simulink model "tester36"  (R2022b)
settings: Solver=VariableStepAuto  StartTime=0.0  StopTime=10  RelTol=1e-3
values from neighbouring files (symbols this model uses):
  IPR = 0.99    [dane.m]    (also in tester23.m; wykresownik33.m; wykresownik35.m; wykresownik36.m)
  P3tDIVP2t_perf = 1.0101    [dane.m]    (also in tester23.m = 1; wykresownik33.m = 1; wykresownik35.m = 1; wykresownik36.m = 1)
  P3tDIVP2t_safe = 1.35    [dane.m]    (also in tester23.m; wykresownik33.m; wykresownik35.m; wykresownik36.m)
libraries: fl_lib x6, nesl_utility x4, SimscapeFluids_lib x3, simulink x1
settings Model: Creator=48519  LastModifiedBy=48519
settings ModelReferenceCC: EnableRefExpFcnMdlSchedulingChecks=on

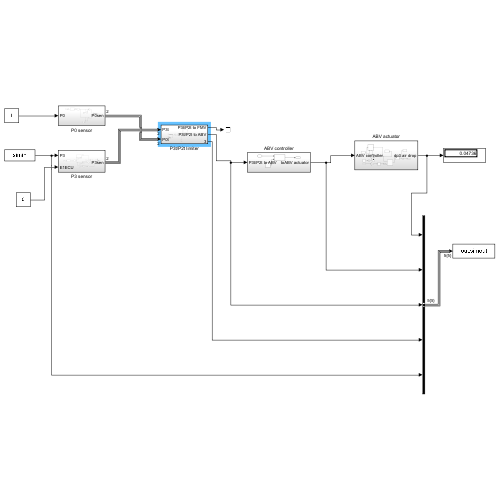
[thumbnail: Simulink's stored preview of the top-level diagram]
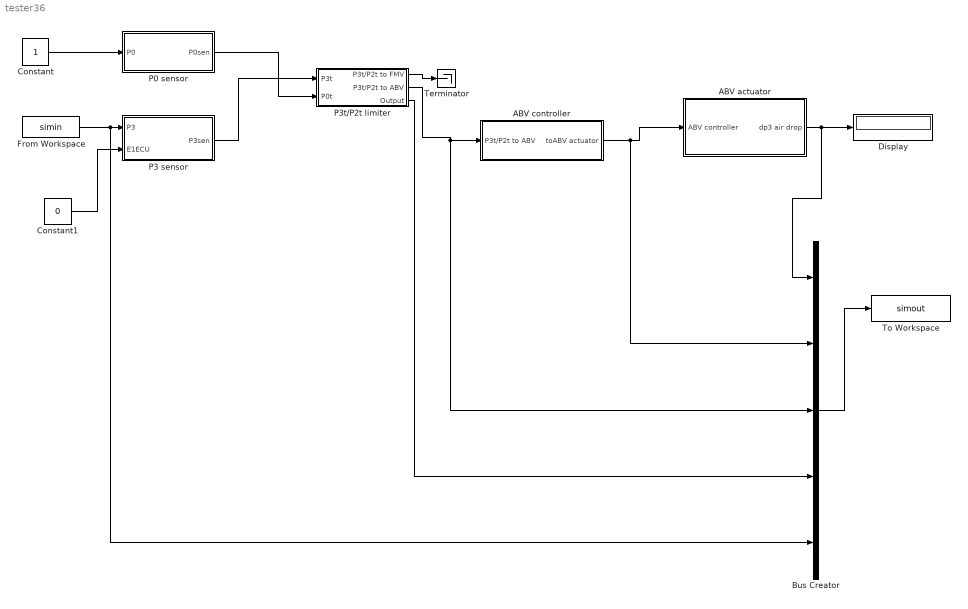
== system tester36 ==
  ABV actuator : Subsystem
  ABV controller : Subsystem
  Bus Creator : BusCreator  Inputs=5
  Constant : Constant
  Constant1 : Constant  Value=0
  Display : Display
  From Workspace : FromWorkspace  VariableName=simin
  P0 sensor : Subsystem
  P3 sensor : Subsystem
  P3t/P2t limiter : Subsystem
  Terminator : Terminator
  To Workspace : ToWorkspace  VariableName=simout  SaveFormat=Timeseries  SampleTime=-1
  wires:
  P3 sensor/1(P3sen) -> P3t/P2t limiter/1(P3t)
  P3t/P2t limiter/1(P3t/P2t to FMV) -> Terminator/1
  P3t/P2t limiter/2(P3t/P2t to ABV) -> Bus Creator/3, ABV controller/1(P3t/P2t to ABV)
  ABV actuator/1(dp3 air drop) -> Bus Creator/1, Display/1
  Constant/1 -> P0 sensor/1(P0)
  From Workspace/1 -> Bus Creator/5, P3 sensor/1(P3)
  Constant1/1 -> P3 sensor/2(E1ECU)
  Bus Creator/1 -> To Workspace/1
  ABV controller/1(toABV actuator) -> Bus Creator/2, ABV actuator/1(ABV controller)
  P3t/P2t limiter/3(Output) -> Bus Creator/4
  P0 sensor/1(P0sen) -> P3t/P2t limiter/2(P0t)

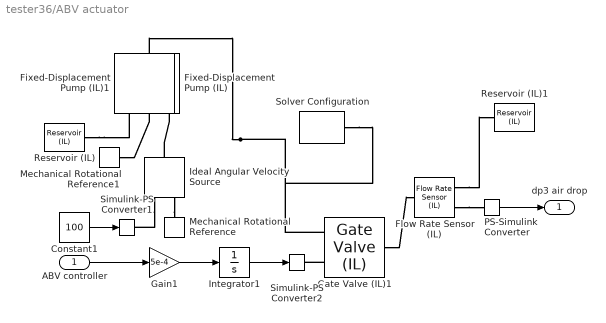
== system tester36/ABV actuator ==
  ABV controller : Inport
  Constant1 : Constant  Value=100
  Fixed-Displacement Pump (IL) : SimscapeFluids_lib/Isothermal Liquid/Pumps & Motors/Fixed-Displacement Pump (IL)  leakage_friction_spec=fluids.isothermal_liquid.pumps_motors.enum.pump_motor_loss_spec.analytical  displacement=30 cm^3/rev  omega_nominal=188 rad/s  p_nominal=10 MPa  vol_eff_nominal=0.92  mech_eff_nominal=0.88  no_load_torque=0 N*m  p_diff_eff_TLU=[.1, 1, 2] MPa  omega_eff_TLU=[25, 50, 100, 200, 300, 400] rad/s  vol_eff_TLU=[.816, .908, .954, .977, .981, .984; .325, .663, .831, .916, .925, .946; .137, .568, .78, .892, .893, .91]  mech_eff_TLU=[.996, .996, .996, .996, .996, .996; .988, .989, .989, .989, .989, .99; .981, .981, .982, .982, .983, .984]  p_diff_loss_TLU=[.1, 1, 2] MPa  omega_loss_TLU=[25, 50, 100, 200, 300, 400] rad/s  vol_loss_TLU=1e-3 * [.023, .023, .023, .023, .0285, .032; .0844, .0842, .0845, .084, .1125, .108; .1079, .108, .11, .108, .1605, .18] m^3/s  mech_loss_TLU=[.002, .002, .002, .002, .002, .002; .0607, .0556, .0556, .0556, .0556, .0505; .1937, .1937, .1833, .1833, .1729, .1626] N*m  vol_eff_min=1e-3  vol_eff_max=1  mech_eff_min=1e-3  mech_eff_max=1  pressure_threshold=1e-3 MPa  omega_threshold=10 rad/s  quadrant_check=simscape.enum.assert.action.none  pump_mode_check=simscape.enum.assert.action.none  pressure_check=simscape.enum.assert.action.none  p_min_valid=0.101325 MPa
      settings: LogSimulationData=on  InternalSimscapePortConfiguration="{\"Bottom\":[{\"id\":\"A\",\"label\":\"A\",\"type\":\"foundation.isothermal_liquid.isothermal_liquid\"}],\"Left\":[],\"Right\":[{\"id\":\"R\",\"label\":\"R\",\"type\":\"foundation.mechanical.rotational.rotational\"},{\"id\":\"C\",\"label\":\"C\",\"type\":\"foundation.mechanical.rotational.rotational\"}],\"Top\":[{\"id\":\"B\",\"label\":\"B\",\"type\":\"foundation.isothermal_liquid.isothermal_liquid\"}]}"
  Fixed-Displacement Pump (IL)1 : SimscapeFluids_lib/Isothermal Liquid/Pumps & Motors/Fixed-Displacement Pump (IL)  leakage_friction_spec=fluids.isothermal_liquid.pumps_motors.enum.pump_motor_loss_spec.analytical  displacement=30 cm^3/rev  omega_nominal=188 rad/s  p_nominal=10 MPa  vol_eff_nominal=0.92  mech_eff_nominal=0.88  no_load_torque=0 N*m  p_diff_eff_TLU=[.1, 1, 2] MPa  omega_eff_TLU=[25, 50, 100, 200, 300, 400] rad/s  vol_eff_TLU=[.816, .908, .954, .977, .981, .984; .325, .663, .831, .916, .925, .946; .137, .568, .78, .892, .893, .91]  mech_eff_TLU=[.996, .996, .996, .996, .996, .996; .988, .989, .989, .989, .989, .99; .981, .981, .982, .982, .983, .984]  p_diff_loss_TLU=[.1, 1, 2] MPa  omega_loss_TLU=[25, 50, 100, 200, 300, 400] rad/s  vol_loss_TLU=1e-3 * [.023, .023, .023, .023, .0285, .032; .0844, .0842, .0845, .084, .1125, .108; .1079, .108, .11, .108, .1605, .18] m^3/s  mech_loss_TLU=[.002, .002, .002, .002, .002, .002; .0607, .0556, .0556, .0556, .0556, .0505; .1937, .1937, .1833, .1833, .1729, .1626] N*m  vol_eff_min=1e-3  vol_eff_max=1  mech_eff_min=1e-3  mech_eff_max=1  pressure_threshold=1e-3 MPa  omega_threshold=10 rad/s  quadrant_check=simscape.enum.assert.action.none  pump_mode_check=simscape.enum.assert.action.none  pressure_check=simscape.enum.assert.action.none  p_min_valid=0.101325 MPa
      settings: LogSimulationData=on  InternalSimscapePortConfiguration="{\"Bottom\":[{\"id\":\"A\",\"label\":\"A\",\"type\":\"foundation.isothermal_liquid.isothermal_liquid\"}],\"Left\":[],\"Right\":[{\"id\":\"R\",\"label\":\"R\",\"type\":\"foundation.mechanical.rotational.rotational\"},{\"id\":\"C\",\"label\":\"C\",\"type\":\"foundation.mechanical.rotational.rotational\"}],\"Top\":[{\"id\":\"B\",\"label\":\"B\",\"type\":\"foundation.isothermal_liquid.isothermal_liquid\"}]}"
  Flow Rate Sensor (IL) : fl_lib/Isothermal Liquid/Sensors/Flow Rate Sensor (IL)  sensor_type=foundation.enum.mass_volumetric_sensor.mass
      settings: InternalSimscapePortConfiguration="{\"Bottom\":[],\"Left\":[{\"id\":\"A\",\"label\":\"A\",\"type\":\"foundation.isothermal_liquid.isothermal_liquid\"}],\"Right\":[{\"id\":\"B\",\"label\":\"B\",\"type\":\"foundation.isothermal_liquid.isothermal_liquid\"},{\"id\":\"M\",\"label\":\"M\",\"type\":\"output\"}],\"Top\":[]}"
  Gain1 : Gain  Gain=5e-4
  Gate Valve (IL)1 : SimscapeFluids_lib/Isothermal Liquid/Valves & Orifices/Flow Control Valves/Gate Valve (IL)  diam_orifice=5.2e-4 m  S_min=0 m  area_leak=1e-100 m^2  area=inf m^2  Cd=0.64  Re_c=150  smoothing_factor=0.01  pressure_recovery=simscape.enum.onoff.off  mdot_A_specify=off  mdot_A_priority=None  mdot_A=0 kg/s  mdot_A_nominal_specify=off  mdot_A_nominal_unit=kg/s  mdot_A_nominal_value=1  mdot_B_specify=off  mdot_B_priority=None  mdot_B=0 kg/s  mdot_B_nominal_specify=off  mdot_B_nominal_unit=kg/s  mdot_B_nominal_value=1
      settings: InternalSimscapePortConfiguration="{\"Bottom\":[],\"Left\":[{\"id\":\"A\",\"label\":\"A\",\"type\":\"foundation.isothermal_liquid.isothermal_liquid\"},{\"id\":\"S\",\"label\":\"S\",\"type\":\"input\"}],\"Right\":[{\"id\":\"B\",\"label\":\"B\",\"type\":\"foundation.isothermal_liquid.isothermal_liquid\"}],\"Top\":[]}"
  Ideal Angular Velocity Source : fl_lib/Mechanical/Mechanical Sources/Ideal Angular Velocity Source
  Integrator1 : Integrator  LimitOutput=on  UpperSaturationLimit=1
  Mechanical Rotational Reference : fl_lib/Mechanical/Rotational Elements/Mechanical Rotational Reference
  Mechanical Rotational Reference1 : fl_lib/Mechanical/Rotational Elements/Mechanical Rotational Reference
  PS-Simulink Converter : nesl_utility/PS-Simulink Converter  PhysicalDomain=network_engine_domain  SubClassName=ps_output  LeftPortType=input  RightPortType=output  PseudoPeriodic=off  Frequencies=[]  VectorFormat=inherit  Unit=inherit  AffineConversion=off
  Reservoir (IL) : fl_lib/Isothermal Liquid/Elements/Reservoir (IL)  reservoir_type=foundation.enum.constant_controlled.constant  pressure_spec=foundation.enum.pressure_spec.atmospheric  reservoir_pressure=0.101325 MPa
  Reservoir (IL)1 : fl_lib/Isothermal Liquid/Elements/Reservoir (IL)  reservoir_type=foundation.enum.constant_controlled.constant  pressure_spec=foundation.enum.pressure_spec.atmospheric  reservoir_pressure=0.101325 MPa
  Simulink-PS Converter1 : nesl_utility/Simulink-PS Converter  PhysicalDomain=network_engine_domain  SubClassName=ps_input  LeftPortType=input  RightPortType=output  PseudoPeriodic=off  Frequencies=[]  NoiseDistribution=none  NoiseParameters=[]  Unit=1  AffineConversion=off  FilteringAndDerivatives=provide  SimscapeFilterOrder=1  InputFilterTimeConstant=0.001  UdotUserProvided=0
  Simulink-PS Converter2 : nesl_utility/Simulink-PS Converter  PhysicalDomain=network_engine_domain  SubClassName=ps_input  LeftPortType=input  RightPortType=output  PseudoPeriodic=off  Frequencies=[]  NoiseDistribution=none  NoiseParameters=[]  Unit=1  AffineConversion=off  FilteringAndDerivatives=provide  SimscapeFilterOrder=1  InputFilterTimeConstant=0.001  UdotUserProvided=0
  Solver Configuration : nesl_utility/Solver Configuration  PhysicalDomain=network_engine_domain  SubClassName=solver  LeftPortType=input  RightPortType=generic  Tones=[]  Harmonics=[]  SimulateNoise=off  Profile=off  UseLocalSampling=off  EnableSwitchedLinearOptims=on  FrequencyDomain=off  UseCCode=off  RelTol=0.001  AbsTol=0.001  MinStep=1e-09  ToWorkspace=off  RevertToSquareIcSolve=off  NumHomotopyIterations=100  PhasorMode=off  PhasorModeNumHarmonics=1  ConsistencySolver=NEWTON_XTOL_AFTER_FTOL  IndexReductionMethod=DerivativeReplacement  DoDC=off  ResidualTolerance=1e-09  ConsistencyTolSource=GLOBAL  ConsistencyAbsTol=0.001  ConsistencyRelTol=0.001  ConsistencyTolFactor=0.001  UseLocalSolver=off  LocalSolverChoice=NE_BACKWARD_EULER_ADVANCER  ResolveIndetEquations=on  FunctionEvalNumThread=1  LocalSolverSampleTime=0.001  DoFixedCost=off  MaxNonlinIter=3  MaxModeIter=2  ComputeImpulses=off  ImpulseIterations=2  LinearAlgebra=auto  LinearAlgebraNumThread=0  EquationFormulation=NE_TIME_EF  DelaysMemoryBudget=1024  AutomaticFiltering=on  FilteringTimeConstant=0.001  PartitionStorageMethod=AS_NEEDED  PartitionMemoryBudget=1024  PartitionMethod=ROBUST
  dp3 air drop : Outport
  wires:
  Integrator1/1 -> Simulink-PS Converter2/1
  Gain1/1 -> Integrator1/1
  Constant1/1 -> Simulink-PS Converter1/1
  ABV controller/1 -> Gain1/1
  PS-Simulink Converter/1 -> dp3 air drop/1
  connections:
  Fixed-Displacement Pump (IL)/LConn1 -- Gate Valve (IL)1/LConn1 -- Solver Configuration/RConn1
  Ideal Angular Velocity Source/LConn1 -- Fixed-Displacement Pump (IL)/RConn1
  Ideal Angular Velocity Source/RConn1 -- Simulink-PS Converter1/RConn1
  Flow Rate Sensor (IL)/RConn1 -- Reservoir (IL)1/LConn1
  Reservoir (IL)/LConn1 -- Fixed-Displacement Pump (IL)/RConn3
  Ideal Angular Velocity Source/RConn2 -- Mechanical Rotational Reference/LConn1
  Flow Rate Sensor (IL)/RConn2 -- PS-Simulink Converter/LConn1
  Gate Valve (IL)1/LConn2 -- Simulink-PS Converter2/RConn1
  Mechanical Rotational Reference1/LConn1 -- Fixed-Displacement Pump (IL)/RConn2
  Gate Valve (IL)1/RConn1 -- Flow Rate Sensor (IL)/LConn1

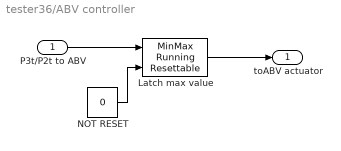
== system tester36/ABV controller ==
  P3t/P2t to ABV : Inport
  Latch max value : simulink/Math Operations/MinMax Running Resettable  Function=max  vinit=0.0
  NOT RESET : Constant  Value=0
  toABV actuator : Outport
  wires:
  P3t/P2t to ABV/1 -> Latch max value/1
  NOT RESET/1 -> Latch max value/2
  Latch max value/1 -> toABV actuator/1

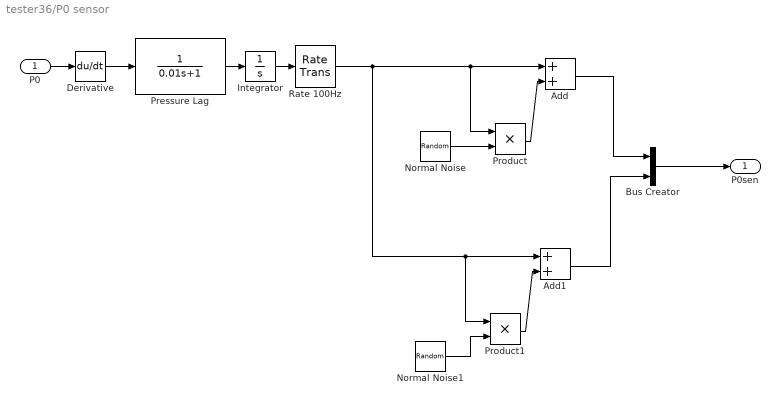
== system tester36/P0 sensor ==
  P0 : Inport
  Add : Sum
  Add1 : Sum
  Bus Creator : BusCreator  Inputs=2
  Derivative : Derivative
  Integrator : Integrator  InitialCondition=1
  Normal Noise : RandomNumber  Variance=((0.005)^2)*pi/2  Seed=31  SampleTime=0.01
  Normal Noise1 : RandomNumber  Variance=((0.005)^2)*pi/2  Seed=33  SampleTime=0.01
  Pressure Lag : TransferFcn  Denominator=[0.01 1]
  Product : Product
  Product1 : Product
  Rate 100Hz : RateTransition  OutPortSampleTimeMultiple=2  OutPortSampleTime=0.01
  P0sen : Outport
  wires:
  P0/1 -> Derivative/1
  Normal Noise1/1 -> Product1/2
  Normal Noise/1 -> Product/2
  Add1/1 -> Bus Creator/2
  Pressure Lag/1 -> Integrator/1
  Bus Creator/1 -> P0sen/1
  Product1/1 -> Add1/2
  Product/1 -> Add/2
  Rate 100Hz/1 -> Add1/1, Product1/1, Add/1, Product/1
  Add/1 -> Bus Creator/1
  Derivative/1 -> Pressure Lag/1
  Integrator/1 -> Rate 100Hz/1

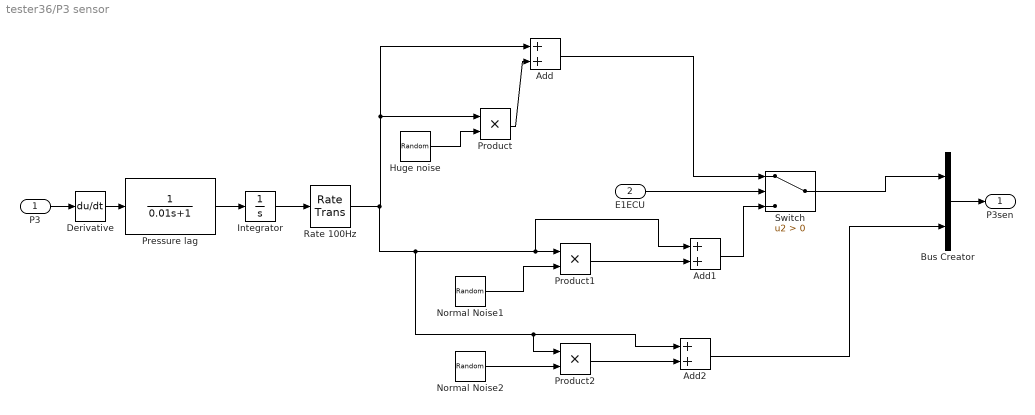
== system tester36/P3 sensor ==
  P3 : Inport
  E1ECU : Inport  Port=2
  Add : Sum
  Add1 : Sum
  Add2 : Sum
  Bus Creator : BusCreator  Inputs=2
  Derivative : Derivative
  Huge noise : RandomNumber  Variance=((0.03)^2)*pi/2  Seed=1  SampleTime=0.01
  Integrator : Integrator  InitialCondition=1
  Normal Noise1 : RandomNumber  Variance=((0.005)^2)*pi/2  Seed=2  SampleTime=0.01
  Normal Noise2 : RandomNumber  Variance=((0.005)^2)*pi/2  Seed=4  SampleTime=0.01
  Pressure lag : TransferFcn  Numerator=[1 ]  Denominator=[0.01 1]
  Product : Product
  Product1 : Product
  Product2 : Product
  Rate 100Hz : RateTransition  OutPortSampleTimeMultiple=2  OutPortSampleTime=0.01
  Switch : Switch  Criteria=u2 > Threshold  SaturateOnIntegerOverflow=off  InputSameDT=off
  P3sen : Outport
  wires:
  Bus Creator/1 -> P3sen/1
  P3/1 -> Derivative/1
  Normal Noise2/1 -> Product2/2
  Add/1 -> Switch/1
  Huge noise/1 -> Product/2
  Add1/1 -> Switch/3
  Product/1 -> Add/2
  Product2/1 -> Add2/2
  Rate 100Hz/1 -> Add2/1, Product2/1, Add1/1, Product1/1, Product/1, Add/1
  Add2/1 -> Bus Creator/2
  Normal Noise1/1 -> Product1/2
  Switch/1 -> Bus Creator/1
  Pressure lag/1 -> Integrator/1
  E1ECU/1 -> Switch/2
  Product1/1 -> Add1/2
  Derivative/1 -> Pressure lag/1
  Integrator/1 -> Rate 100Hz/1

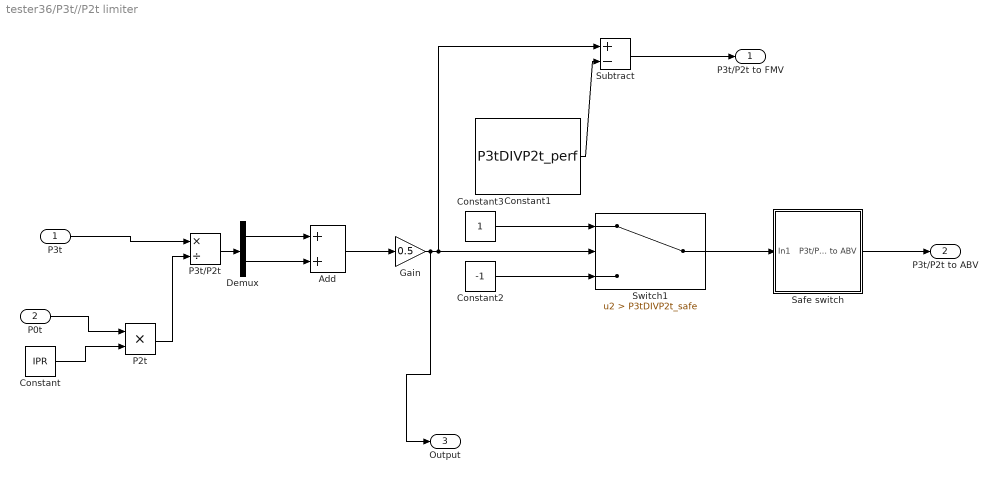
== system tester36/P3t//P2t limiter ==
  P3t : Inport
  P0t : Inport  Port=2
  Add : Sum
  Constant : Constant  Value=IPR
  Constant1 : Constant  Value=P3tDIVP2t_perf
  Constant2 : Constant  Value=-1
  Constant3 : Constant
  Demux : Demux  Outputs=2
  Gain : Gain  Gain=0.5
  P2t : Product
  P3t/P2t : Product  Inputs=*/
  Safe switch : Subsystem
  Subtract : Sum  Inputs=+-
  Switch1 : Switch  Criteria=u2 > Threshold  Threshold=P3tDIVP2t_safe  SaturateOnIntegerOverflow=off  InputSameDT=off
  P3t/P2t to FMV : Outport
  P3t/P2t to ABV : Outport  Port=2
  Output : Outport  Port=3
  wires:
  Subtract/1 -> P3t/P2t to FMV/1
  P3t/1 -> P3t/P2t/1
  Constant1/1 -> Subtract/2
  Gain/1 -> Output/1, Switch1/2, Subtract/1
  Constant2/1 -> Switch1/3
  Switch1/1 -> Safe switch/1(In1)
  Constant3/1 -> Switch1/1
  Demux/2 -> Add/2
  Demux/1 -> Add/1
  Add/1 -> Gain/1
  P3t/P2t/1 -> Demux/1
  Safe switch/1(P3t/P2t to ABV) -> P3t/P2t to ABV/1
  Constant/1 -> P2t/2
  P2t/1 -> P3t/P2t/2
  P0t/1 -> P2t/1

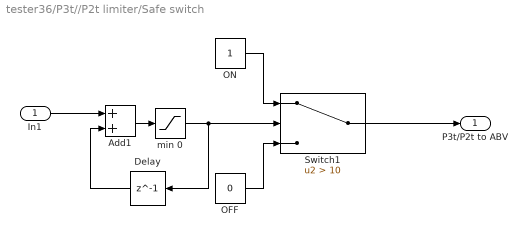
== system tester36/P3t//P2t limiter/Safe switch ==
  In1 : Inport
  Add1 : Sum
  Delay : Delay  DelayLength=1
  OFF : Constant  Value=0
  ON : Constant
  Switch1 : Switch  Criteria=u2 > Threshold  Threshold=10  SaturateOnIntegerOverflow=off  InputSameDT=off
  min 0 : Saturate  UpperLimit=100  LowerLimit=0
  P3t/P2t to ABV : Outport
  wires:
  ON/1 -> Switch1/1
  Delay/1 -> Add1/2
  Add1/1 -> min 0/1
  Switch1/1 -> P3t/P2t to ABV/1
  min 0/1 -> Switch1/2, Delay/1
  OFF/1 -> Switch1/3
  In1/1 -> Add1/1
